simulink model "LAB1_4_sim"  (R2025b)
settings: Solver=VariableStepAuto  StartTime=0.0  StopTime=10.0  RelTol=1e-3
undefined symbols (not defined in the file or in its folder): Beq, daq, degs2rpm, delta_c, drv, gbox, Jeq, k_z0, k_z1, k_z2, k_zx, mot, pulse2deg, rads2rpm, Req, rpm2rads, Tausf, w0, w_c
settings Model: Creator=Gioele  LastModifiedBy=Simone

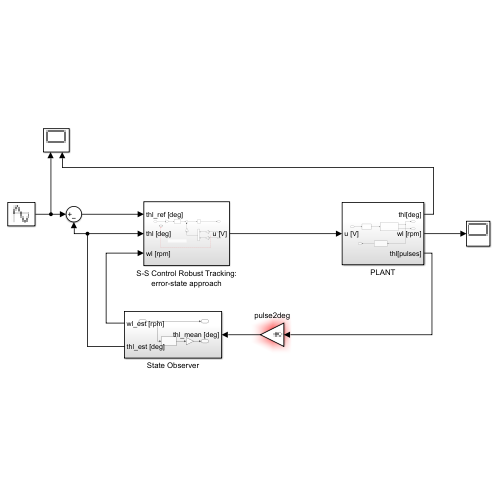
[thumbnail: Simulink's stored preview of the top-level diagram]
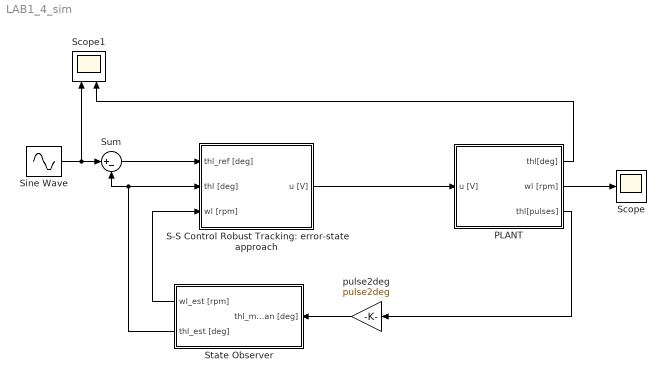
== system LAB1_4_sim ==
  PLANT : Subsystem
  S-S Control Robust Tracking: error-state approach : Subsystem
  Scope : Scope
      settings: ActiveDisplayYMinimum=-1  ActiveDisplayYMaximum=1
  Scope1 : Scope  NumInputPorts=2
      settings: ActiveDisplayYMinimum=-63.08  ActiveDisplayYMaximum=65.8771
  Sine Wave : Sin  Amplitude=40  Frequency=10  SampleTime=0
  State Observer : Subsystem
  Sum : Sum  Inputs=|+-
  pulse2deg : Gain  Gain=pulse2deg
  wires:
  pulse2deg/1 -> State Observer/1(thl_mean [deg])
  State Observer/2(thl_est [deg]) -> Sum/2, S-S Control Robust Tracking: error-state approach/2(thl [deg])
  State Observer/1(wl_est [rpm]) -> S-S Control Robust Tracking: error-state approach/3(wl [rpm])
  Sine Wave/1 -> Sum/1, Scope1/1
  Sum/1 -> S-S Control Robust Tracking: error-state approach/1(thl_ref [deg])
  S-S Control Robust Tracking: error-state approach/1(u [V]) -> PLANT/1(u [V])
  PLANT/1(thl[deg]) -> Scope1/2
  PLANT/2(wl [rpm]) -> Scope/1
  PLANT/3(thl[pulses]) -> pulse2deg/1

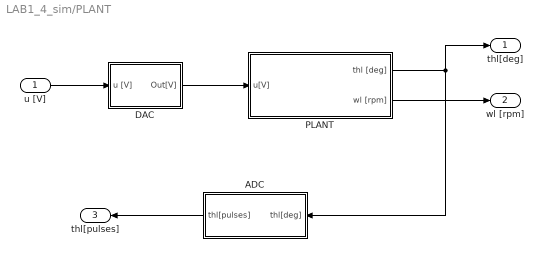
== system LAB1_4_sim/PLANT ==
  u [V] : Inport
  ADC : Subsystem  TreatAsAtomicUnit=on
  DAC : Subsystem  TreatAsAtomicUnit=on
  PLANT : Subsystem
  thl[deg] : Outport
  wl [rpm] : Outport  Port=2
  thl[pulses] : Outport  Port=3
  wires:
  ADC/1(thl[pulses]) -> thl[pulses]/1
  DAC/1(Out[V]) -> PLANT/1(u[V])
  PLANT/1(thl [deg]) -> thl[deg]/1, ADC/1(thl[deg])
  PLANT/2(wl [rpm]) -> wl [rpm]/1
  u [V]/1 -> DAC/1(u [V])

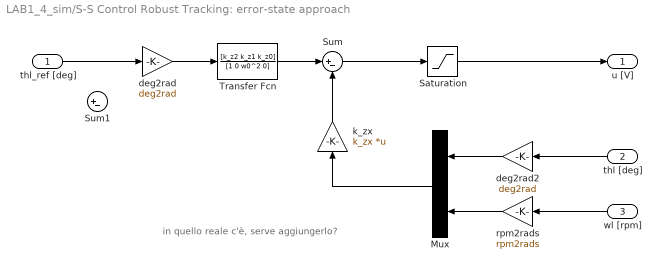
== system LAB1_4_sim/S-S Control Robust Tracking: error-state approach ==
  note: in quello reale c'è, serve aggiungerlo?
  thl_ref [deg] : Inport
  thl [deg] : Inport  Port=2
  wl [rpm] : Inport  Port=3
  Mux : Mux  Inputs=2
  Saturation : Saturate  UpperLimit=10  LowerLimit=-10  ZeroCross=off
  Sum : Sum  Inputs=|+-
  Sum1 : Sum  Inputs=|+-
  Transfer Fcn : TransferFcn  Numerator=[k_z2 k_z1 k_z0]  Denominator=[1 0 w0^2 0]
  deg2rad : Gain  Gain=deg2rad
  deg2rad2 : Gain  Gain=deg2rad
  k_zx : Gain  Gain=k_zx  Multiplication=Matrix(K*u)
  rpm2rads : Gain  Gain=rpm2rads
  u [V] : Outport
  wires:
  deg2rad2/1 -> Mux/1
  rpm2rads/1 -> Mux/2
  thl_ref [deg]/1 -> deg2rad/1
  Saturation/1 -> u [V]/1
  thl [deg]/1 -> deg2rad2/1
  wl [rpm]/1 -> rpm2rads/1
  Mux/1 -> k_zx/1
  k_zx/1 -> Sum/2
  Sum/1 -> Saturation/1
  deg2rad/1 -> Transfer Fcn/1
  Transfer Fcn/1 -> Sum/1
  ? -> Sum1/2

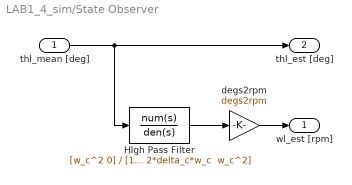
== system LAB1_4_sim/State Observer ==
  thl_mean [deg] : Inport
  HIgh Pass Filter : TransferFcn  Numerator=[w_c^2 0]  Denominator="[1 2*delta_c*w_c  w_c^2]"
  degs2rpm : Gain  Gain=degs2rpm
  wl_est [rpm] : Outport
  thl_est [deg] : Outport  Port=2
  wires:
  thl_mean [deg]/1 -> HIgh Pass Filter/1, thl_est [deg]/1
  HIgh Pass Filter/1 -> degs2rpm/1
  degs2rpm/1 -> wl_est [rpm]/1

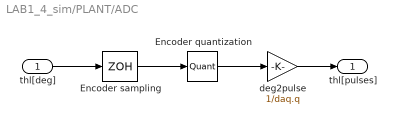
== system LAB1_4_sim/PLANT/ADC ==
  thl[deg] : Inport
  Encoder quantization : Quantizer  QuantizationInterval=daq.q
  Encoder sampling : ZeroOrderHold  SampleTime=daq.dac.Ts
  deg2pulse : Gain  Gain=1/daq.q
  thl[pulses] : Outport
  wires:
  Encoder quantization/1 -> deg2pulse/1
  thl[deg]/1 -> Encoder sampling/1
  Encoder sampling/1 -> Encoder quantization/1
  deg2pulse/1 -> thl[pulses]/1

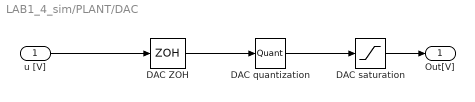
== system LAB1_4_sim/PLANT/DAC ==
  u [V] : Inport
  "DAC ZOH " : ZeroOrderHold  SampleTime=daq.dac.Ts
  DAC quantization : Quantizer  QuantizationInterval=daq.dac.q
  DAC saturation : Saturate  UpperLimit=daq.dac.fs  LowerLimit=-daq.dac.fs
  Out[V] : Outport
  wires:
  DAC quantization/1 -> DAC saturation/1
  u [V]/1 -> "DAC ZOH "/1
  "DAC ZOH "/1 -> DAC quantization/1
  DAC saturation/1 -> Out[V]/1

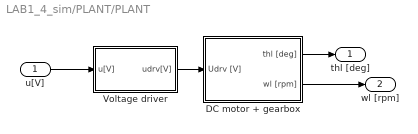
== system LAB1_4_sim/PLANT/PLANT ==
  u[V] : Inport
  DC motor + gearbox : Subsystem
  Voltage driver : Subsystem  TreatAsAtomicUnit=on
  thl [deg] : Outport
  wl [rpm] : Outport  Port=2
  wires:
  Voltage driver/1(udrv[V]) -> DC motor + gearbox/1(Udrv [V])
  DC motor + gearbox/2(wl [rpm]) -> wl [rpm]/1
  DC motor + gearbox/1(thl [deg]) -> thl [deg]/1
  u[V]/1 -> Voltage driver/1(u[V])

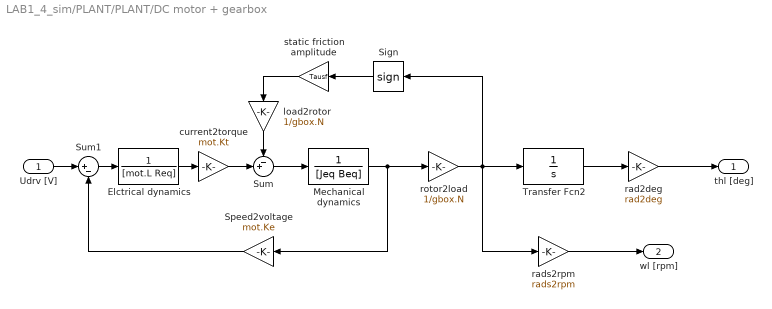
== system LAB1_4_sim/PLANT/PLANT/DC motor + gearbox ==
  Udrv [V] : Inport
  Elctrical dynamics : TransferFcn  Denominator=[mot.L Req]
  Mechanical dynamics : TransferFcn  Denominator=[Jeq Beq]
  Sign : Signum  ZeroCross=off
  Speed2voltage : Gain  Gain=mot.Ke
  Sum : Sum  Inputs=-+|
  Sum1 : Sum  Inputs=|+-
  Transfer Fcn2 : TransferFcn  Denominator=[1 0]
  current2torque : Gain  Gain=mot.Kt
  load2rotor : Gain  Gain=1/gbox.N
  rad2deg : Gain  Gain=rad2deg
  rads2rpm : Gain  Gain=rads2rpm
  rotor2load : Gain  Gain=1/gbox.N
  static friction amplitude : Gain  Gain=Tausf
  thl [deg] : Outport
  wl [rpm] : Outport  Port=2
  wires:
  rotor2load/1 -> Sign/1, rads2rpm/1, Transfer Fcn2/1
  Sign/1 -> static friction amplitude/1
  rads2rpm/1 -> wl [rpm]/1
  Sum/1 -> Mechanical dynamics/1
  Udrv [V]/1 -> Sum1/1
  static friction amplitude/1 -> load2rotor/1
  load2rotor/1 -> Sum/1
  Transfer Fcn2/1 -> rad2deg/1
  current2torque/1 -> Sum/2
  Speed2voltage/1 -> Sum1/2
  Mechanical dynamics/1 -> Speed2voltage/1, rotor2load/1
  Elctrical dynamics/1 -> current2torque/1
  Sum1/1 -> Elctrical dynamics/1
  rad2deg/1 -> thl [deg]/1

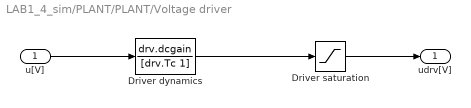
== system LAB1_4_sim/PLANT/PLANT/Voltage driver ==
  u[V] : Inport  OutMax=[5]
  Driver dynamics : TransferFcn  Numerator=drv.dcgain  Denominator=[drv.Tc 1]
  Driver saturation : Saturate  UpperLimit=drv.outmax  LowerLimit=-drv.outmax
  udrv[V] : Outport
  wires:
  Driver dynamics/1 -> Driver saturation/1
  u[V]/1 -> Driver dynamics/1
  Driver saturation/1 -> udrv[V]/1
